simulink model "control_core"  (R2022b)
settings: Solver=FixedStepAuto  StartTime=0.0  StopTime=60  FixedStep=.01  RelTol=1e-3
undefined symbols (not defined in the file): CdProp, Ct, Earth, g, Ixx, Iyy, Izz, larm, mass, WGS84
libraries: slpidlib x6, sharedtransform x4, simulink x2, aerolibutil x2, aerolibtransform2 x1, shared6dof x1, aerolibfltsims x1, vrlib x1
(part 1 of 2)
settings Model: Creator=aaron  LastModifiedBy=aaron
settings DebuggingCC: ModelReferenceExtraNoncontSigs=none

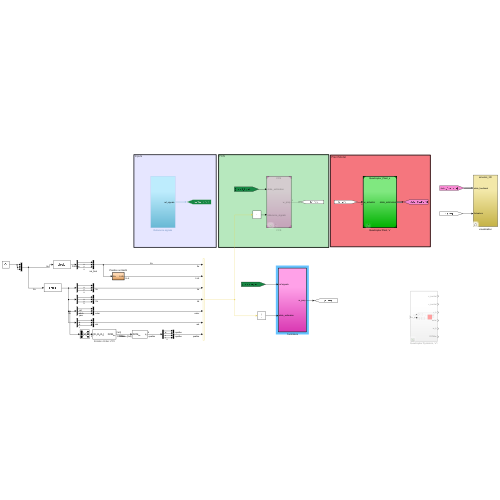
[thumbnail: Simulink's stored preview of the top-level diagram]
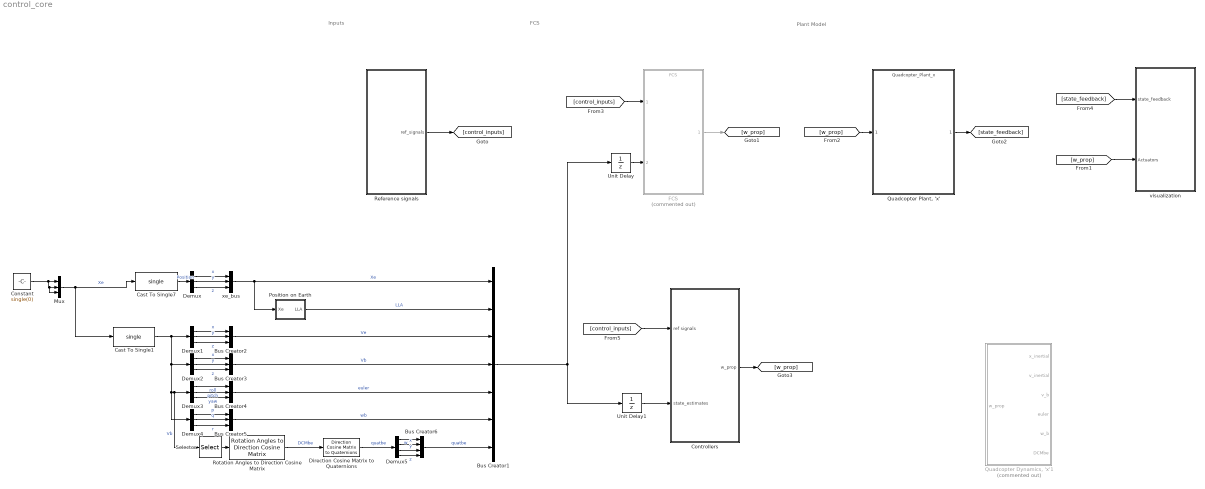
== system control_core ==
  note: Plant Model
  note: Inputs
  note: FCS
  Bus Creator1 : BusCreator  Inputs=7  OutDataTypeStr=Bus: state_estimates
  Bus Creator2 : BusCreator  Inputs=3  OutDataTypeStr=Bus: Velocity
  Bus Creator3 : BusCreator  Inputs=3  OutDataTypeStr=Bus: Velocity
  Bus Creator4 : BusCreator  Inputs=3  OutDataTypeStr=Bus: euler
  Bus Creator5 : BusCreator  Inputs=3  OutDataTypeStr=Bus: body_rates
  Bus Creator6 : BusCreator  Inputs=4  OutDataTypeStr=Bus: quat
  Cast To Single1 : DataTypeConversion  OutDataTypeStr=single  SaturateOnIntegerOverflow=off  RndMeth=Floor
  Cast To Single7 : DataTypeConversion  OutDataTypeStr=single  SaturateOnIntegerOverflow=off  RndMeth=Floor
  Constant : Constant  Value=single(0)  OutDataTypeStr=single
  Controllers : Subsystem  TreatAsAtomicUnit=on
  Demux{,1..4} (5 alike) : Demux  Outputs=3
  Demux5 : Demux
  Direction Cosine Matrix to Quaternions : sharedtransform/Direction Cosine Matrix  to Quaternions  aMode=0  action=None  tolerance=eps(2)
      settings: LibrarySourceBlock=|
      | aerolibtransform2/Direction Cosine Matrix
      | to Quaternions
  FCS : ModelReference  Commented=on  ModelNameDialog=FCS  SimulationMode=Normal  ModelReferenceVersion=1.59
  Mux : Mux  Inputs=3
  Position on Earth : Subsystem  Priority=1  TreatAsAtomicUnit=on
  "Quadcopter Dynamics, 'x'1" : Subsystem  Commented=on
  "Quadcopter Plant, 'x'" : ModelReference  ModelNameDialog=Quadcopter_Plant_x  SimulationMode=Normal  ModelReferenceVersion=1.62
  Reference signals : Subsystem
  Rotation Angles to Direction Cosine Matrix : sharedtransform/Rotation Angles to Direction Cosine Matrix  rotationOrder=ZYX  aMode=aMode
  Selector : Selector  InputPortWidth=3  IndexOptions=Index vector (dialog)  Indices=[3 2 1]  OutputSizes=1
  Unit Delay : UnitDelay  SampleTime=-1  HasFrameUpgradeWarning=on
  Unit Delay1 : UnitDelay  SampleTime=-1  HasFrameUpgradeWarning=on
  visualization : Subsystem  Variant=on  VariantControl=Choice
  xe_bus : BusCreator  Inputs=3  OutDataTypeStr=Bus: Position
  wires:
  FCS/1 -> [w_prop]
  Bus Creator1/1 -> Unit Delay/1, Unit Delay1/1
  Unit Delay/1 -> FCS/2
  [w_prop] -> visualization/2(Actuators)
  [w_prop] -> "Quadcopter Plant, 'x'"/1
  Reference signals/1(ref_signals) -> [control_inputs]
  [control_inputs] -> FCS/1
  "Quadcopter Plant, 'x'"/1 -> [state_feedback]
  [state_feedback] -> visualization/1(state_feedback)
  Demux4/2 -> Bus Creator5/2  "q"
  Demux5/4 -> Bus Creator6/4  "z"
  Demux/2 -> xe_bus/2  "y"
  Demux/3 -> xe_bus/3  "z"
  xe_bus/1 -> Bus Creator1/1, Position on Earth/1(Xe)  "Xe"
  Bus Creator4/1 -> Bus Creator1/5  "euler"
  Direction Cosine Matrix to Quaternions/1 -> Demux5/1  "quatbe"
  Demux/1 -> xe_bus/1  "x"
  Demux1/3 -> Bus Creator2/3  "z"
  Demux1/2 -> Bus Creator2/2  "y"
  Demux1/1 -> Bus Creator2/1  "x"
  Demux3/1 -> Bus Creator4/1  "roll"
  Demux3/2 -> Bus Creator4/2  "pitch"
  Demux3/3 -> Bus Creator4/3  "yaw"
  Bus Creator2/1 -> Bus Creator1/3  "Ve"
  Demux2/2 -> Bus Creator3/2  "y"
  Demux2/1 -> Bus Creator3/1  "x"
  Mux/1 -> Cast To Single1/1, Cast To Single7/1  "Xe"
  Demux4/1 -> Bus Creator5/1  "p"
  Bus Creator5/1 -> Bus Creator1/6  "wb"
  Bus Creator6/1 -> Bus Creator1/7  "quatbe"
  Demux2/3 -> Bus Creator3/3  "z"
  Demux5/3 -> Bus Creator6/3  "y"
  Bus Creator3/1 -> Bus Creator1/4  "Vb"
  Demux4/3 -> Bus Creator5/3  "r"
  Rotation Angles to Direction Cosine Matrix/1 -> Direction Cosine Matrix to Quaternions/1  "DCMbe"
  Selector/1 -> Rotation Angles to Direction Cosine Matrix/1
  Position on Earth/1(LLA) -> Bus Creator1/2  "LLA"
  Demux5/1 -> Bus Creator6/1  "w"
  Demux5/2 -> Bus Creator6/2  "x"
  Constant/1 -> Mux/3, Mux/2, Mux/1
  Cast To Single7/1 -> Demux/1  "Position"
  Cast To Single1/1 -> Demux4/1, Selector/1, Demux3/1, Demux2/1, Demux1/1  "Vb"
  [control_inputs] -> Controllers/1(ref signals)
  Unit Delay1/1 -> Controllers/2(state_estimates)
  Controllers/1(w_prop) -> [w_prop]

== system control_core/Controllers ==
  ref signals : Inport  OutDataTypeStr=Bus: reference_signals  LockScale=on
  state_estimates : Inport  Port=2  OutDataTypeStr=Bus: state_estimates  LockScale=on
  Flight Controller : Subsystem
  Motor Mixing : Subsystem
  w_prop : Outport
  wires:
  state_estimates/1 -> Flight Controller/2(state_estimates)
  Flight Controller/1(Force command) -> Motor Mixing/1(Force)
  Motor Mixing/1(motor_rpm) -> w_prop/1  "w_prop"
  Flight Controller/2(Torque command) -> Motor Mixing/2(Torque)
  ref signals/1 -> Flight Controller/1(ref signals)

== system control_core/Position on Earth ==
  Xe : Inport  OutDataTypeStr=Bus: Position  Unit=m
  Bus Creator : BusCreator  Inputs=3  OutDataTypeStr=Bus: LLA
  Bus Selector : BusSelector  OutputSignals=x,y,z  OutputAsBus=on
  Bus to Vector : BusToVector
  Cast To Single : DataTypeConversion  OutDataTypeStr=single  SaturateOnIntegerOverflow=off  RndMeth=Floor
  Cast To Single1 : DataTypeConversion  OutDataTypeStr=single  SaturateOnIntegerOverflow=off  RndMeth=Floor
  Demux : Demux  Outputs=2
  Flat Earth to LLA : aerolibtransform2/Flat Earth to LLA  units=Metric (MKS)  ptype=Earth (WGS84)  F=1/298.257223563  R=6378137  refPosPort=off  LL0=[-122.389977, 37.615223]  psi=0
  href : Constant  Value=-4
  LLA : Outport  OutDataTypeStr=Bus: LLA  VectorParamsAs1DForOutWhenUnconnected=off
  wires:
  Bus Creator/1 -> LLA/1
  href/1 -> Flat Earth to LLA/2
  Demux/2 -> Bus Creator/2  "long"
  Flat Earth to LLA/1 -> Cast To Single/1
  Demux/1 -> Bus Creator/1  "lat"
  Flat Earth to LLA/2 -> Cast To Single1/1  "altitude"
  Xe/1 -> Bus Selector/1
  Bus Selector/1 -> Bus to Vector/1
  Bus to Vector/1 -> Flat Earth to LLA/1
  Cast To Single/1 -> Demux/1
  Cast To Single1/1 -> Bus Creator/3  "altitude"

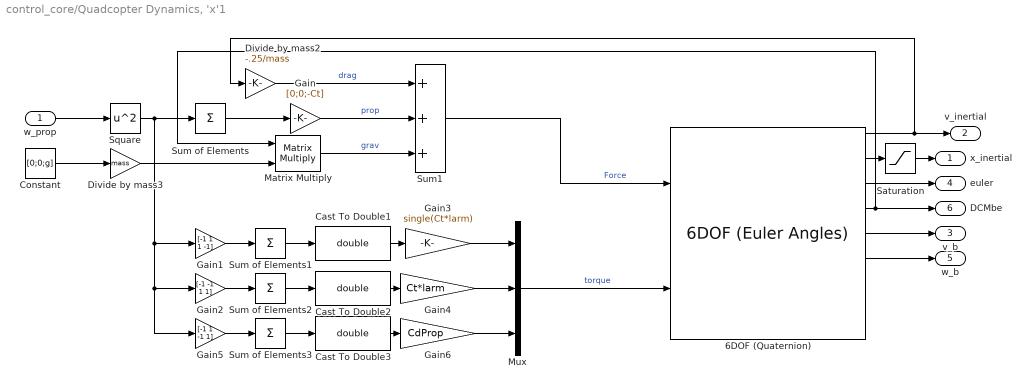
== system control_core/Quadcopter Dynamics, 'x'1 ==
  w_prop : Inport
  6DOF (Quaternion) : shared6dof/6DOF (Euler Angles)  units=Metric (MKS)  mtype=Fixed  rep=Euler Angles  xme_0=[0,0,0]  Vm_0=[0,0,0]  eul_0=[0,0,0]  pm_0=[0,0,0]  mass_0=mass  mass_e=0.5  mass_f=2.0  inertia=diag([Ixx Iyy Izz])  inertia_e=eye(3)  inertia_f=2*eye(3)  k_quat=Vehicle.SixDOF.quatGain  vre_flag=on  abi_flag=on  aMode=aMode  xme_statename=''  Vm_statename=''  eul_statename=''  quat_statename=''  pm_statename=''  mass_statename=''
  Cast To Double1 : DataTypeConversion  OutDataTypeStr=double  SaturateOnIntegerOverflow=off  RndMeth=Floor
  Cast To Double2 : DataTypeConversion  OutDataTypeStr=double  SaturateOnIntegerOverflow=off  RndMeth=Floor
  Cast To Double3 : DataTypeConversion  OutDataTypeStr=double  SaturateOnIntegerOverflow=off  RndMeth=Floor
  Constant : Constant  Value=[0;0;g]
  Divide by mass2 : Gain  Gain=-.25/mass
  Divide by mass3 : Gain  Gain=mass
  Gain : Gain  Gain=[0;0;-Ct]
  Gain1 : Gain  Gain=[-1 1 1 -1]
  Gain2 : Gain  Gain=[-1 -1 1 1]
  Gain3 : Gain  Gain=single(Ct*larm)
  Gain4 : Gain  Gain=Ct*larm
  Gain5 : Gain  Gain=[-1 1 -1 1]
  Gain6 : Gain  Gain=CdProp
  Matrix Multiply : Product  Multiplication=Matrix(*)
  Mux : Mux  Inputs=3
  Saturation : Saturate  UpperLimit=[inf inf 0]  LowerLimit=-inf
  Square : Math  Operator=square
  Sum of Elements{,1..3} (4 alike) : Sum  Inputs=+
  Sum1 : Sum  Inputs=+++
  x_inertial : Outport
  v_inertial : Outport  Port=2
  v_b : Outport  Port=3
  euler : Outport  Port=4
  w_b : Outport  Port=5
  DCMbe : Outport  Port=6
  wires:
  Sum1/1 -> 6DOF (Quaternion)/1  "Force"
  Constant/1 -> Divide by mass3/1
  6DOF (Quaternion)/1 -> v_inertial/1, Divide by mass2/1
  Divide by mass2/1 -> Sum1/1  "drag"
  w_prop/1 -> Square/1
  Square/1 -> Gain5/1, Gain2/1, Gain1/1, Sum of Elements/1
  Sum of Elements/1 -> Gain/1
  Gain/1 -> Sum1/2  "prop"
  Gain1/1 -> Sum of Elements1/1
  Gain2/1 -> Sum of Elements2/1
  Gain5/1 -> Sum of Elements3/1
  Gain3/1 -> Mux/1
  Gain4/1 -> Mux/2
  Gain6/1 -> Mux/3
  Mux/1 -> 6DOF (Quaternion)/2  "torque"
  6DOF (Quaternion)/5 -> v_b/1
  6DOF (Quaternion)/2 -> Saturation/1
  6DOF (Quaternion)/6 -> w_b/1
  6DOF (Quaternion)/3 -> euler/1
  6DOF (Quaternion)/4 -> Matrix Multiply/1, DCMbe/1
  Cast To Double1/1 -> Gain3/1
  Sum of Elements1/1 -> Cast To Double1/1
  Cast To Double2/1 -> Gain4/1
  Sum of Elements2/1 -> Cast To Double2/1
  Sum of Elements3/1 -> Cast To Double3/1
  Cast To Double3/1 -> Gain6/1
  Saturation/1 -> x_inertial/1
  Divide by mass3/1 -> Matrix Multiply/2
  Matrix Multiply/1 -> Sum1/3  "grav"

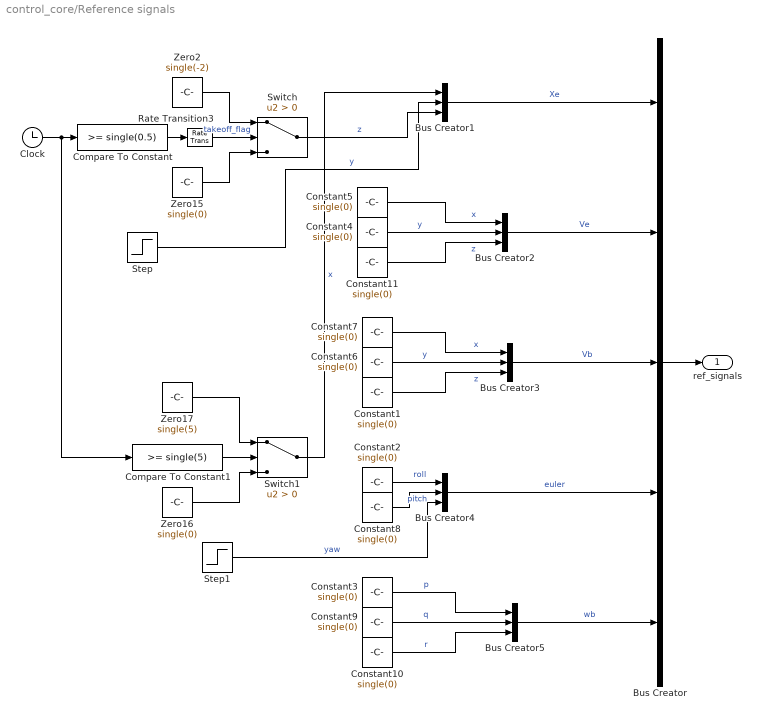
== system control_core/Reference signals ==
  Bus Creator : BusCreator  Inputs=5  OutDataTypeStr=Bus: reference_signals
      settings: InheritFromInputs=off
  Bus Creator1 : BusCreator  Inputs=3  OutDataTypeStr=Bus: Position
  Bus Creator2 : BusCreator  Inputs=3  OutDataTypeStr=Bus: Velocity
  Bus Creator3 : BusCreator  Inputs=3  OutDataTypeStr=Bus: Velocity
  Bus Creator4 : BusCreator  Inputs=3  OutDataTypeStr=Bus: euler
  Bus Creator5 : BusCreator  Inputs=3  OutDataTypeStr=Bus: body_rates
  Clock : Clock
  Compare To Constant : simulink/Logic and Bit Operations/Compare To Constant  relop=>=  const=single(0.5)  OutDataTypeStr=boolean
  Compare To Constant1 : simulink/Logic and Bit Operations/Compare To Constant  relop=>=  const=single(5)  OutDataTypeStr=boolean
  Constant{1..11} (11 alike) : Constant  Value=single(0)  OutDataTypeStr=single
  Rate Transition3 : RateTransition  OutPortSampleTime=.01
  Step : Step  Time=10  After=single(5)  OutDataTypeStr=single  SampleTime=0
  Step1 : Step  Time=10  After=single(pi/2)  OutDataTypeStr=single  SampleTime=0
  Switch : Switch  Criteria=u2 > Threshold  SaturateOnIntegerOverflow=off  InputSameDT=off
  Switch1 : Switch  Criteria=u2 > Threshold  SaturateOnIntegerOverflow=off  InputSameDT=off
  Zero15 : Constant  Value=single(0)  OutDataTypeStr=single
  Zero16 : Constant  Value=single(0)  OutDataTypeStr=single
  Zero17 : Constant  Value=single(5)  OutDataTypeStr=single
  Zero2 : Constant  Value=single(-2)  OutDataTypeStr=single
  ref_signals : Outport  OutDataTypeStr=Bus: reference_signals  SampleTime=.01  LockScale=on
  wires:
  Bus Creator4/1 -> Bus Creator/4  "euler"
  Bus Creator1/1 -> Bus Creator/1  "Xe"
  Bus Creator2/1 -> Bus Creator/2  "Ve"
  Bus Creator/1 -> ref_signals/1
  Zero15/1 -> Switch/3
  Zero2/1 -> Switch/1
  Clock/1 -> Compare To Constant1/1, Compare To Constant/1
  Compare To Constant/1 -> Rate Transition3/1
  Rate Transition3/1 -> Switch/2  "takeoff_flag"
  Compare To Constant1/1 -> Switch1/2
  Zero16/1 -> Switch1/3
  Zero17/1 -> Switch1/1
  Switch/1 -> Bus Creator1/3  "z"
  Step/1 -> Bus Creator1/2  "y"
  Step1/1 -> Bus Creator4/3  "yaw"
  Switch1/1 -> Bus Creator1/1  "x"
  Constant2/1 -> Bus Creator4/1  "roll"
  Constant5/1 -> Bus Creator2/1  "x"
  Constant4/1 -> Bus Creator2/2  "y"
  Constant11/1 -> Bus Creator2/3  "z"
  Constant7/1 -> Bus Creator3/1  "x"
  Bus Creator3/1 -> Bus Creator/3  "Vb"
  Constant6/1 -> Bus Creator3/2  "y"
  Constant1/1 -> Bus Creator3/3  "z"
  Constant8/1 -> Bus Creator4/2  "pitch"
  Constant9/1 -> Bus Creator5/2  "q"
  Constant10/1 -> Bus Creator5/3  "r"
  Bus Creator5/1 -> Bus Creator/5  "wb"
  Constant3/1 -> Bus Creator5/1  "p"

== system control_core/visualization ==
  state_feedback : Inport  OutDataTypeStr=Bus: state_estimates
  Actuators : Inport  Port=2
  flight_gear : Subsystem  VariantControl=sim_3D == 0
  simulink_3D : Subsystem  VariantControl=sim_3D == 1

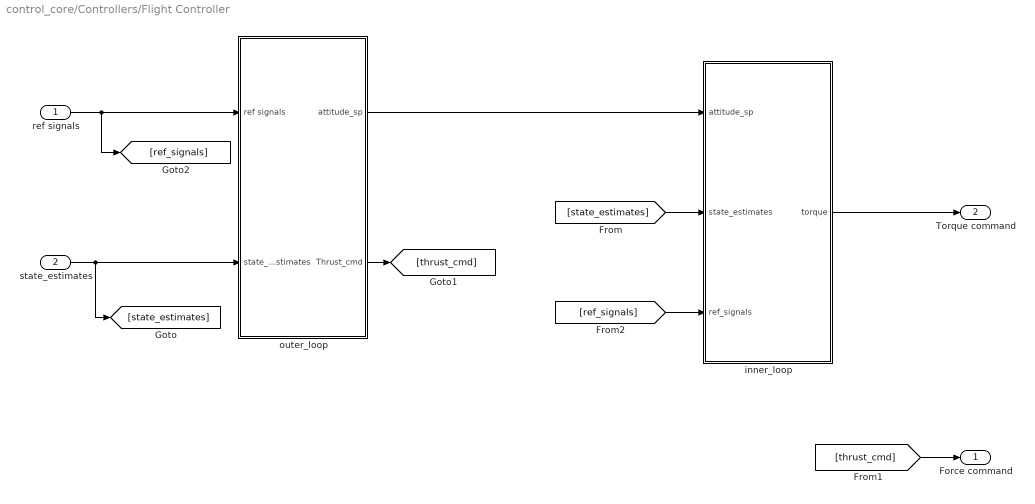
== system control_core/Controllers/Flight Controller ==
  ref signals : Inport  OutDataTypeStr=Bus: reference_signals  LockScale=on
  state_estimates : Inport  Port=2  OutDataTypeStr=Bus: state_estimates  LockScale=on
  inner_loop : Subsystem
  outer_loop : Subsystem
  Force command : Outport
  Torque command : Outport  Port=2
  wires:
  [ref_signals] -> inner_loop/3(ref_signals)
  [thrust_cmd] -> Force command/1
  outer_loop/2(Thrust_cmd) -> [thrust_cmd]
  inner_loop/1(torque) -> Torque command/1
  [state_estimates] -> inner_loop/2(state_estimates)
  outer_loop/1(attitude_sp) -> inner_loop/1(attitude_sp)
  ref signals/1 -> outer_loop/1(ref signals), [ref_signals]
  state_estimates/1 -> [state_estimates], outer_loop/2(state_estimates)

== system control_core/Controllers/Motor Mixing ==
  Force : Inport
  Torque : Inport  Port=2
  Cast To Single : DataTypeConversion  OutDataTypeStr=single  SaturateOnIntegerOverflow=off  RndMeth=Floor
  MATLAB Function : MATLAB Function  TreatAsAtomicUnit=on
  Matrix Multiply : Product  Multiplication=Matrix(*)
  Mux : Mux  Inputs=2
  Saturation : Saturate  UpperLimit=2000  LowerLimit=0
  SignedSqrt1 : Sqrt  Operator=signedSqrt  IntermediateResultsDataTypeStr=single
  motor_rpm : Outport
  wires:
  Mux/1 -> Cast To Single/1
  Cast To Single/1 -> Matrix Multiply/2
  MATLAB Function/1(controlMatInv) -> Matrix Multiply/1  "invcontrolMat"
  Matrix Multiply/1 -> SignedSqrt1/1
  SignedSqrt1/1 -> Saturation/1
  Saturation/1 -> motor_rpm/1
  Force/1 -> Mux/1
  Torque/1 -> Mux/2  "torque"

== system control_core/visualization/flight_gear ==
  state_feedback : Inport  OutDataTypeStr=Bus: state_estimates
  Actuators : Inport  Port=2
  Flight_gear : Subsystem
  wires:
  state_feedback/1 -> [state_feedback]
  [state_feedback] -> Flight_gear/1(state_feedback)
  Actuators/1 -> [actuators]

== system control_core/visualization/simulink_3D ==
  state_feedback : Inport  OutDataTypeStr=Bus: state_estimates
  Actuators : Inport  Port=2
  Simulink 3D : Subsystem  VariantControl=VSS_VISUALIZATION==VisualizationMode.Simulink_3D
  wires:
  state_feedback/1 -> [state_feedback]
  [state_feedback] -> Simulink 3D/1(state_feedback)
  Actuators/1 -> [actuators]
  [actuators] -> Simulink 3D/2(Actuators)

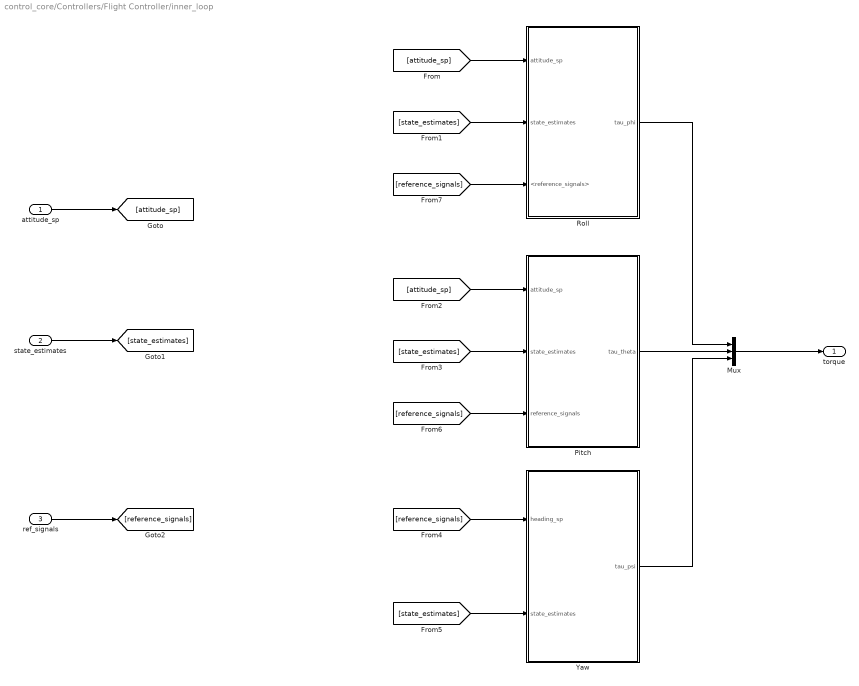
== system control_core/Controllers/Flight Controller/inner_loop ==
  attitude_sp : Inport
  state_estimates : Inport  Port=2  OutDataTypeStr=Bus: state_estimates
  ref_signals : Inport  Port=3  OutDataTypeStr=Bus: reference_signals
  Mux : Mux  Inputs=3
  Pitch : Subsystem
  Roll : Subsystem
  Yaw : Subsystem
  torque : Outport
  wires:
  Yaw/1(tau_psi) -> Mux/3
  Pitch/1(tau_theta) -> Mux/2
  Mux/1 -> torque/1
  Roll/1(tau_phi) -> Mux/1
  [state_estimates] -> Yaw/2(state_estimates)
  [state_estimates] -> Pitch/2(state_estimates)
  [attitude_sp] -> Pitch/1(attitude_sp)
  [state_estimates] -> Roll/2(state_estimates)
  [attitude_sp] -> Roll/1(attitude_sp)
  state_estimates/1 -> [state_estimates]
  attitude_sp/1 -> [attitude_sp]
  ref_signals/1 -> [reference_signals]
  [reference_signals] -> Yaw/1(heading_sp)
  [reference_signals] -> Pitch/3(reference_signals)
  [reference_signals] -> Roll/3(<reference_signals>)

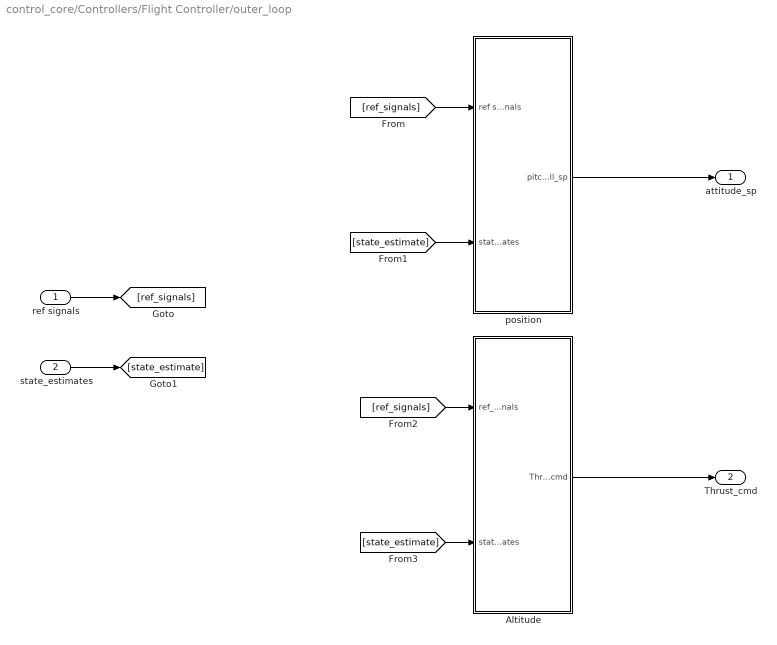
== system control_core/Controllers/Flight Controller/outer_loop ==
  ref signals : Inport  OutDataTypeStr=Bus: reference_signals  LockScale=on
  state_estimates : Inport  Port=2  OutDataTypeStr=Bus: state_estimates  LockScale=on
  Altitude : Subsystem
  position : Subsystem
  attitude_sp : Outport
  Thrust_cmd : Outport  Port=2
  wires:
  [state_estimate] -> Altitude/2(state_estimates)
  [ref_signals] -> Altitude/1(ref_signals)
  [state_estimate] -> position/2(state_estimates)
  [ref_signals] -> position/1(ref signals)
  state_estimates/1 -> [state_estimate]
  ref signals/1 -> [ref_signals]
  Altitude/1(Thrust_cmd) -> Thrust_cmd/1
  position/1(pitch_roll_sp) -> attitude_sp/1

== system control_core/visualization/flight_gear/Flight_gear ==
  state_feedback : Inport  OutDataTypeStr=Bus: state_estimates
  Bus Selector : BusSelector  OutputSignals=LLA,euler
  Demux5 : Demux  Outputs=3
  FlightGear Preconfigured 6DoF Animation : aerolibfltsims/FlightGear Preconfigured 6DoF Animation  Commented=on  xFlightGearVersion=v2019.1  DestinationIpAddress=127.0.0.1  DestinationPort=5502  SampleTime=.0001  packetVersion=24
  Mux1 : Mux  Inputs=2
  Mux2 : Mux  Inputs=3
  Transpose : Math  Operator=transpose
  wires:
  Demux5/3 -> Mux2/3
  Mux2/1 -> Transpose/1
  Demux5/2 -> Mux2/1
  Mux1/1 -> FlightGear Preconfigured 6DoF Animation/1
  Bus Selector/2 -> Mux1/2  "<euler>"
  Demux5/1 -> Mux2/2
  Transpose/1 -> Mux1/1
  Bus Selector/1 -> Demux5/1  "<LLA>"
  state_feedback/1 -> Bus Selector/1

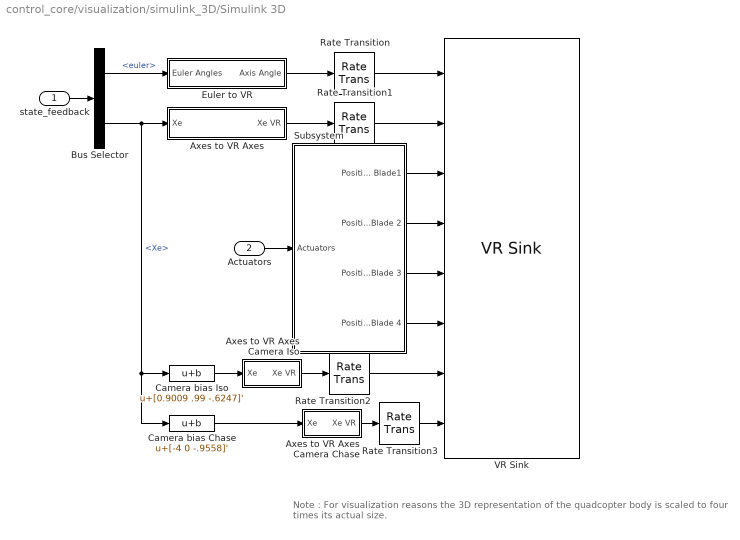
== system control_core/visualization/simulink_3D/Simulink 3D ==
  note: Note : For visualization reasons the 3D representation of the quadcopter body is scaled to four times its actual size.
  state_feedback : Inport  OutDataTypeStr=Bus: state_estimates
  Actuators : Inport  Port=2
  Axes to VR Axes : Subsystem
  Axes to VR Axes Camera Chase : Subsystem
  Axes to VR Axes Camera Iso : Subsystem
  Bus Selector : BusSelector  OutputSignals=euler,Xe
  Camera bias Chase : Bias  Bias=[-4 0 -.9558]'  SaturateOnIntegerOverflow=off
  Camera bias Iso : Bias  Bias=[0.9009 .99 -.6247]'  SaturateOnIntegerOverflow=off
  Euler to VR : Subsystem
  Rate Transition{,1..3} (4 alike) : RateTransition
  Subsystem : Subsystem
  VR Sink : vrlib/VR Sink  InstantiateOnLoad=on  SampleTime=10*.01  ViewEnable=on  RemoteChange=off  RemoteView=off  FieldsWritten=QuadBody.rotation.4.1.1.double#QuadBody.translation.3.1.1.double#Blade1.rotation.4.1.1.double#Blade2.rotation.4.1.1.double#Blade3.rotation.4.1.1.double#Blade4.rotation.4.1.1.double#IsoNoRotation.position.3.1.1.double#OnQuadNoRotation.position.3.1.1.double  WorldFileName=asbQuadcopterWorld.wrl  AutoView=on  VideoDimensions=[]  AllowVariableSize=off  FigureProperties="{'Position', 'Name', 'Viewpoint', 'CameraBound', 'CameraDirection', 'CameraPosition', 'CameraUpVector', 'ZoomFactor', 'Antialiasing', 'Headlight', 'Lighting', 'NavPanel', 'Sound', 'StatusBar', 'Stereo3D', 'Stereo3DCameraOffset', 'Stereo3DHIT', 'ToolBar', 'Textures', 'Transparency', 'Triad', 'Wireframe', 'NavZones', 'NavMode', 'NavSpeed', 'CaptureFileFormat', 'CaptureFileName', 'Record2DCompressMethod', 'Record2DCompressQuality', 'Record2D', 'Record2DFileName', 'Record2DFPS'; [5.0000000000000000e+00   9.2000000000000000e+01   5.7600000000000000e+02   3.5000000000000000e+02], '', 'Isometric', 'on', [0.0000000000000000e+00   0.0000000000000000e+00  -1.0000000000000000e+00], [0.0000000000000000e+00   0.0000000000000000e+00   0.0000000000000000e+00], [0.0000000000000000e+00   1.0000000000000000e+00   0.0000000000000000e+00], [1.0000000000000000e+00], 'off', 'on', 'on', 'halfbar', 'on', 'on', 'off', [1.0000000149011612e-01], [0.0000000000000000e+00], 'on', 'on', 'on', 'none', 'off', 'off', 'fly', 'normal', 'tif', '%f_anim_%n.tif', 'auto', [7.5000000000000000e+01], 'off', '%f_anim_%n.avi', 'auto'}"
  wires:
  Euler to VR/1(Axis Angle) -> Rate Transition/1
  Axes to VR Axes/1(Xe VR) -> Rate Transition1/1
  Bus Selector/1 -> Euler to VR/1(Euler Angles)  "<euler>"
  Bus Selector/2 -> Axes to VR Axes/1(Xe), Camera bias Chase/1, Camera bias Iso/1  "<Xe>"
  state_feedback/1 -> Bus Selector/1
  Actuators/1 -> Subsystem/1(Actuators)
  Axes to VR Axes Camera Iso/1(Xe VR) -> Rate Transition2/1
  Camera bias Iso/1 -> Axes to VR Axes Camera Iso/1(Xe)
  Rate Transition/1 -> VR Sink/1
  Rate Transition1/1 -> VR Sink/2
  Subsystem/1(Position Blade1) -> VR Sink/3
  Subsystem/2(Position Blade 2) -> VR Sink/4
  Subsystem/3(Position Blade 3) -> VR Sink/5
  Subsystem/4(Position Blade 4) -> VR Sink/6
  Rate Transition2/1 -> VR Sink/7
  Axes to VR Axes Camera Chase/1(Xe VR) -> Rate Transition3/1
  Rate Transition3/1 -> VR Sink/8
  Camera bias Chase/1 -> Axes to VR Axes Camera Chase/1(Xe)

== system control_core/Controllers/Flight Controller/inner_loop/Pitch ==
  attitude_sp : Inport
  state_estimates : Inport  Port=2  OutDataTypeStr=Bus: state_estimates
  reference_signals : Inport  Port=3  OutDataTypeStr=Bus: reference_signals
  Bus Selector : BusSelector  OutputSignals=euler.pitch
  PID Controller : slpidlib/PID Controller  Controller=PID  Form=Parallel  TimeDomain=Discrete-time  UseExternalTs=off  SampleTime=-1  IntegratorMethod=Forward Euler  FilterMethod=Forward Euler  ControllerParametersSource=internal  P=0.000755  I=1.95e-05  UseKiTs=off  D=0.00509  N=1.0382  UseFilter=on  TunerSelectOption=Transfer Function Based (PID Tuner App)  InitialConditionSource=internal  InitialConditionForIntegrator=0  InitialConditionForFilter=0  DifferentiatorICPrevScaledInput=0  ExternalReset=none  TrackingMode=off  Kt=1  LimitOutput=off  SatLimitsSource=internal  UpperSaturationLimit=inf  LowerSaturationLimit=-inf  LinearizeAsGain=on  AntiWindupMode=clamping  Kb=1  LimitIntegrator=off  UpperIntegratorSaturationLimit=inf  LowerIntegratorSaturationLimit=-inf  POutMin=[]  POutMax=[]  IOutMin=[]  IOutMax=[]  DOutMin=[]  DOutMax=[]  NOutMin=[]  NOutMax=[]  SumOutMin=[]  SumOutMax=[]  SaturationOutMin=[]  SaturationOutMax=[]  PParamMin=[]  PParamMax=[]  IParamMin=[]  IParamMax=[]  DParamMin=[]  DParamMax=[]  NParamMin=[]  NParamMax=[]  KbParamMin=[]  KbParamMax=[]  KtParamMin=[]  KtParamMax=[]  KbOutMin=[]  KbOutMax=[]  KtOutMin=[]  KtOutMax=[]  IntegratorOutMin=[]  IntegratorOutMax=[]  FilterOutMin=[]  FilterOutMax=[]  SumI1OutMin=[]  SumI1OutMax=[]  SumI2OutMin=[]  SumI2OutMax=[]  SumI3OutMin=[]  SumI3OutMax=[]  SumI4OutMin=[]  SumI4OutMax=[]  SumDOutMin=[]  SumDOutMax=[]  DifferentiatorOutMin=[]  DifferentiatorOutMax=[]  FilterDiffOutCoefMin=[]  FilterDiffOutCoefMax=[]  ReciprocalOutMin=[]  ReciprocalOutMax=[]  SumDenOutMin=[]  SumDenOutMax=[]  SumNumOutMin=[]  SumNumOutMax=[]  DivideOutMin=[]  DivideOutMax=[]  UdiffTsProdOutMin=[]  UdiffTsProdOutMax=[]  NTsProdOutMin=[]  NTsProdOutMax=[]  UintegralTsProdOutMin=[]  UintegralTsProdOutMax=[]  UngainTsProdOutMin=[]  UngainTsProdOutMax=[]  ClampingZeroOutDataTypeStr=Inherit: Inherit via back propagation  ClampingZeroOutMin=[]  ClampingZeroOutMax=[]  FilterDenConstantOutDataTypeStr=Inherit: Inherit via back propagation  FilterDenConstantOutMin=[]  FilterDenConstantOutMax=[]  PCopyOutDataTypeStr=Inherit: Inherit via back propagation  PCopyOutMin=[]  PCopyOutMax=[]  NCopyOutDataTypeStr=Inherit: Inherit via back propagation  NCopyOutMin=[]  NCopyOutMax=[]  IntegratorContinuousStateAttributes=''  IntegratorStateMustResolveToSignalObject=off  IntegratorRTWStateStorageClass=Auto  FilterContinuousStateAttributes=''  FilterStateMustResolveToSignalObject=off  FilterRTWStateStorageClass=Auto  ParallelPVariant=InternalParameters  IdealPVariant=Disabled  IVariant=InternalParameters  DVariant=InternalParameters  IntegratorVariant=Discrete  SatVariant=Disabled  AWVariant=Passthrough  PCopyVariant=Disabled  TRVariant=Disabled  FdbkBlocksVariant=Forward  IdealPFdbkVariant=Disabled  SatFdbkVariant=Disabled  DerivativeFilterVariant=ForwardEulerFilter  NVariant=InternalParameters  NCopyVariant=Disabled  FilterICVariant=InternalICsFilter  IntegratorICVariant=InternalICs  ExternalResetVariant=Disabled  TRSumVariant=Passthrough  SumFdbkVariant=Disabled  SumVariant=Sum_PID  TsampFilterVariant=InternalTs  TsampNgainVariant=Passthrough  TsampIntegralVariant=Passthrough  ExternalSaturationOutDataTypeStr=Inherit: Same as second input
  Selector : Selector  InputPortWidth=2  IndexOptions=Index vector (dialog)  Indices=[2]  OutputSizes=1
  Sum : Sum  Inputs=|+-
  Terminator : Terminator
  tau_theta : Outport
  wires:
  Selector/1 -> Sum/1
  reference_signals/1 -> Terminator/1
  state_estimates/1 -> Bus Selector/1
  Bus Selector/1 -> Sum/2  "<pitch>"
  PID Controller/1 -> tau_theta/1
  Sum/1 -> PID Controller/1
  attitude_sp/1 -> Selector/1

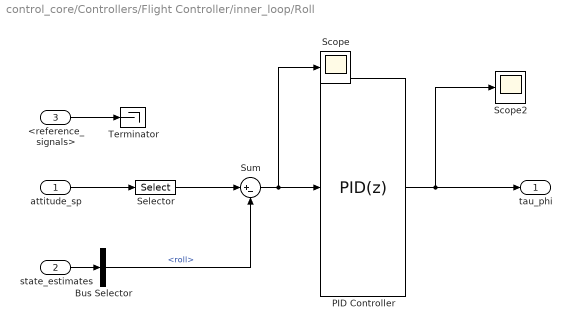
== system control_core/Controllers/Flight Controller/inner_loop/Roll ==
  attitude_sp : Inport
  state_estimates : Inport  Port=2  OutDataTypeStr=Bus: state_estimates
  <reference_signals> : Inport  Port=3  OutDataTypeStr=Bus: reference_signals
  Bus Selector : BusSelector  OutputSignals=euler.roll
  PID Controller : slpidlib/PID Controller  Controller=PID  Form=Parallel  TimeDomain=Discrete-time  UseExternalTs=off  SampleTime=-1  IntegratorMethod=Forward Euler  FilterMethod=Forward Euler  ControllerParametersSource=internal  P=0.00222776202264695  I=2.18485015437245e-05  UseKiTs=off  D=0.0134340999324703  N=1.24748629813611  UseFilter=on  TunerSelectOption=Transfer Function Based (PID Tuner App)  InitialConditionSource=internal  InitialConditionForIntegrator=0  InitialConditionForFilter=0  DifferentiatorICPrevScaledInput=0  ExternalReset=none  TrackingMode=off  Kt=1  LimitOutput=off  SatLimitsSource=internal  UpperSaturationLimit=inf  LowerSaturationLimit=-inf  LinearizeAsGain=on  AntiWindupMode=clamping  Kb=1  LimitIntegrator=off  UpperIntegratorSaturationLimit=inf  LowerIntegratorSaturationLimit=-inf  POutMin=[]  POutMax=[]  IOutMin=[]  IOutMax=[]  DOutMin=[]  DOutMax=[]  NOutMin=[]  NOutMax=[]  SumOutMin=[]  SumOutMax=[]  SaturationOutMin=[]  SaturationOutMax=[]  PParamMin=[]  PParamMax=[]  IParamMin=[]  IParamMax=[]  DParamMin=[]  DParamMax=[]  NParamMin=[]  NParamMax=[]  KbParamMin=[]  KbParamMax=[]  KtParamMin=[]  KtParamMax=[]  KbOutMin=[]  KbOutMax=[]  KtOutMin=[]  KtOutMax=[]  IntegratorOutMin=[]  IntegratorOutMax=[]  FilterOutMin=[]  FilterOutMax=[]  SumI1OutMin=[]  SumI1OutMax=[]  SumI2OutMin=[]  SumI2OutMax=[]  SumI3OutMin=[]  SumI3OutMax=[]  SumI4OutMin=[]  SumI4OutMax=[]  SumDOutMin=[]  SumDOutMax=[]  DifferentiatorOutMin=[]  DifferentiatorOutMax=[]  FilterDiffOutCoefMin=[]  FilterDiffOutCoefMax=[]  ReciprocalOutMin=[]  ReciprocalOutMax=[]  SumDenOutMin=[]  SumDenOutMax=[]  SumNumOutMin=[]  SumNumOutMax=[]  DivideOutMin=[]  DivideOutMax=[]  UdiffTsProdOutMin=[]  UdiffTsProdOutMax=[]  NTsProdOutMin=[]  NTsProdOutMax=[]  UintegralTsProdOutMin=[]  UintegralTsProdOutMax=[]  UngainTsProdOutMin=[]  UngainTsProdOutMax=[]  ClampingZeroOutDataTypeStr=Inherit: Inherit via back propagation  ClampingZeroOutMin=[]  ClampingZeroOutMax=[]  FilterDenConstantOutDataTypeStr=Inherit: Inherit via back propagation  FilterDenConstantOutMin=[]  FilterDenConstantOutMax=[]  PCopyOutDataTypeStr=Inherit: Inherit via back propagation  PCopyOutMin=[]  PCopyOutMax=[]  NCopyOutDataTypeStr=Inherit: Inherit via back propagation  NCopyOutMin=[]  NCopyOutMax=[]  IntegratorContinuousStateAttributes=''  IntegratorStateMustResolveToSignalObject=off  IntegratorRTWStateStorageClass=Auto  FilterContinuousStateAttributes=''  FilterStateMustResolveToSignalObject=off  FilterRTWStateStorageClass=Auto  ParallelPVariant=InternalParameters  IdealPVariant=Disabled  IVariant=InternalParameters  DVariant=InternalParameters  IntegratorVariant=Discrete  SatVariant=Disabled  AWVariant=Passthrough  PCopyVariant=Disabled  TRVariant=Disabled  FdbkBlocksVariant=Forward  IdealPFdbkVariant=Disabled  SatFdbkVariant=Disabled  DerivativeFilterVariant=ForwardEulerFilter  NVariant=InternalParameters  NCopyVariant=Disabled  FilterICVariant=InternalICsFilter  IntegratorICVariant=InternalICs  ExternalResetVariant=Disabled  TRSumVariant=Passthrough  SumFdbkVariant=Disabled  SumVariant=Sum_PID  TsampFilterVariant=InternalTs  TsampNgainVariant=Passthrough  TsampIntegralVariant=Passthrough  ExternalSaturationOutDataTypeStr=Inherit: Same as second input
  Scope : Scope
  Scope2 : Scope
  Selector : Selector  InputPortWidth=2  IndexOptions=Index vector (dialog)  Indices=[1]  OutputSizes=1
  Sum : Sum  Inputs=|+-
  Terminator : Terminator
  tau_phi : Outport
  wires:
  Selector/1 -> Sum/1
  <reference_signals>/1 -> Terminator/1
  Bus Selector/1 -> Sum/2  "<roll>"
  state_estimates/1 -> Bus Selector/1
  PID Controller/1 -> tau_phi/1, Scope2/1
  Sum/1 -> Scope/1, PID Controller/1
  attitude_sp/1 -> Selector/1

== system control_core/Controllers/Flight Controller/inner_loop/Yaw ==
  heading_sp : Inport  OutDataTypeStr=Bus: reference_signals
  state_estimates : Inport  Port=2  OutDataTypeStr=Bus: state_estimates
  Bus Selector : BusSelector  OutputSignals=euler.yaw
  Bus Selector1 : BusSelector  OutputSignals=euler.yaw
  PID Controller : slpidlib/PID Controller  Controller=PD  Form=Parallel  TimeDomain=Discrete-time  UseExternalTs=off  SampleTime=-1  IntegratorMethod=Forward Euler  FilterMethod=Forward Euler  ControllerParametersSource=internal  P=0.00308709400862221  I=0  UseKiTs=off  D=0.020762699011989  N=9.31948574377754  UseFilter=on  TunerSelectOption=Transfer Function Based (PID Tuner App)  InitialConditionSource=internal  InitialConditionForIntegrator=0  InitialConditionForFilter=0  DifferentiatorICPrevScaledInput=0  ExternalReset=none  TrackingMode=off  Kt=1  LimitOutput=off  SatLimitsSource=internal  UpperSaturationLimit=inf  LowerSaturationLimit=-inf  LinearizeAsGain=on  AntiWindupMode=clamping  Kb=1  LimitIntegrator=off  UpperIntegratorSaturationLimit=inf  LowerIntegratorSaturationLimit=-inf  POutMin=[]  POutMax=[]  IOutMin=[]  IOutMax=[]  DOutMin=[]  DOutMax=[]  NOutMin=[]  NOutMax=[]  SumOutMin=[]  SumOutMax=[]  SaturationOutMin=[]  SaturationOutMax=[]  PParamMin=[]  PParamMax=[]  IParamMin=[]  IParamMax=[]  DParamMin=[]  DParamMax=[]  NParamMin=[]  NParamMax=[]  KbParamMin=[]  KbParamMax=[]  KtParamMin=[]  KtParamMax=[]  KbOutMin=[]  KbOutMax=[]  KtOutMin=[]  KtOutMax=[]  IntegratorOutMin=[]  IntegratorOutMax=[]  FilterOutMin=[]  FilterOutMax=[]  SumI1OutMin=[]  SumI1OutMax=[]  SumI2OutMin=[]  SumI2OutMax=[]  SumI3OutMin=[]  SumI3OutMax=[]  SumI4OutMin=[]  SumI4OutMax=[]  SumDOutMin=[]  SumDOutMax=[]  DifferentiatorOutMin=[]  DifferentiatorOutMax=[]  FilterDiffOutCoefMin=[]  FilterDiffOutCoefMax=[]  ReciprocalOutMin=[]  ReciprocalOutMax=[]  SumDenOutMin=[]  SumDenOutMax=[]  SumNumOutMin=[]  SumNumOutMax=[]  DivideOutMin=[]  DivideOutMax=[]  UdiffTsProdOutMin=[]  UdiffTsProdOutMax=[]  NTsProdOutMin=[]  NTsProdOutMax=[]  UintegralTsProdOutMin=[]  UintegralTsProdOutMax=[]  UngainTsProdOutMin=[]  UngainTsProdOutMax=[]  ClampingZeroOutDataTypeStr=Inherit: Inherit via back propagation  ClampingZeroOutMin=[]  ClampingZeroOutMax=[]  FilterDenConstantOutDataTypeStr=Inherit: Inherit via back propagation  FilterDenConstantOutMin=[]  FilterDenConstantOutMax=[]  PCopyOutDataTypeStr=Inherit: Inherit via back propagation  PCopyOutMin=[]  PCopyOutMax=[]  NCopyOutDataTypeStr=Inherit: Inherit via back propagation  NCopyOutMin=[]  NCopyOutMax=[]  IntegratorContinuousStateAttributes=''  IntegratorStateMustResolveToSignalObject=off  IntegratorRTWStateStorageClass=Auto  FilterContinuousStateAttributes=''  FilterStateMustResolveToSignalObject=off  FilterRTWStateStorageClass=Auto  ParallelPVariant=InternalParameters  IdealPVariant=Disabled  IVariant=Disabled  DVariant=InternalParameters  IntegratorVariant=Disabled  SatVariant=Disabled  AWVariant=Disabled  PCopyVariant=Disabled  TRVariant=Disabled  FdbkBlocksVariant=Forward  IdealPFdbkVariant=Disabled  SatFdbkVariant=Disabled  DerivativeFilterVariant=ForwardEulerFilter  NVariant=InternalParameters  NCopyVariant=Disabled  FilterICVariant=InternalICsFilter  IntegratorICVariant=Disabled  ExternalResetVariant=Disabled  TRSumVariant=Passthrough  SumFdbkVariant=Disabled  SumVariant=Sum_PD  TsampFilterVariant=InternalTs  TsampNgainVariant=Passthrough  TsampIntegralVariant=Disabled_SignalSpec  ExternalSaturationOutDataTypeStr=Inherit: Same as second input
  Sum : Sum  Inputs=|+-
  tau_psi : Outport
  wires:
  Sum/1 -> PID Controller/1
  state_estimates/1 -> Bus Selector/1
  Bus Selector/1 -> Sum/2  "<yaw>"
  PID Controller/1 -> tau_psi/1
  Bus Selector1/1 -> Sum/1  "<yaw>"
  heading_sp/1 -> Bus Selector1/1  "heading_sp"

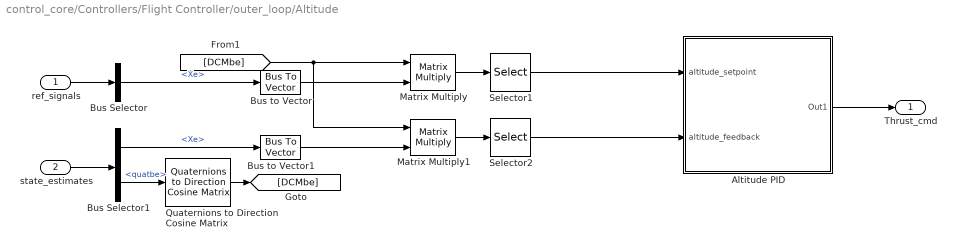
== system control_core/Controllers/Flight Controller/outer_loop/Altitude ==
  ref_signals : Inport  OutDataTypeStr=Bus: reference_signals
  state_estimates : Inport  Port=2  OutDataTypeStr=Bus: state_estimates
  Altitude PID : Subsystem
  Bus Selector : BusSelector  OutputSignals=Xe
  Bus Selector1 : BusSelector  OutputSignals=Xe,quatbe
  Bus to Vector : BusToVector
  Bus to Vector1 : BusToVector
  Matrix Multiply : Product  Multiplication=Matrix(*)
  Matrix Multiply1 : Product  Multiplication=Matrix(*)
  Quaternions to Direction Cosine Matrix : sharedtransform/Quaternions to  Direction Cosine Matrix  aMode=aMode
      settings: LibrarySourceBlock=|
      | aerolibtransform2/Quaternions to
      | Direction Cosine Matrix
  Selector1 : Selector  InputPortWidth=3  IndexOptions=Index vector (dialog)  Indices=[3]  OutputSizes=1
  Selector2 : Selector  InputPortWidth=3  IndexOptions=Index vector (dialog)  Indices=[3]  OutputSizes=1
  Thrust_cmd : Outport
  wires:
  Altitude PID/1(Out1) -> Thrust_cmd/1
  Selector2/1 -> Altitude PID/2(altitude_feedback)
  Selector1/1 -> Altitude PID/1(altitude_setpoint)
  Matrix Multiply/1 -> Selector1/1
  Matrix Multiply1/1 -> Selector2/1
  [DCMbe] -> Matrix Multiply/1, Matrix Multiply1/1
  Bus Selector1/2 -> Quaternions to Direction Cosine Matrix/1  "<quatbe>"
  state_estimates/1 -> Bus Selector1/1
  ref_signals/1 -> Bus Selector/1
  Bus Selector/1 -> Bus to Vector/1  "<Xe>"
  Bus Selector1/1 -> Bus to Vector1/1  "<Xe>"
  Bus to Vector/1 -> Matrix Multiply/2
  Bus to Vector1/1 -> Matrix Multiply1/2
  Quaternions to Direction Cosine Matrix/1 -> [DCMbe]

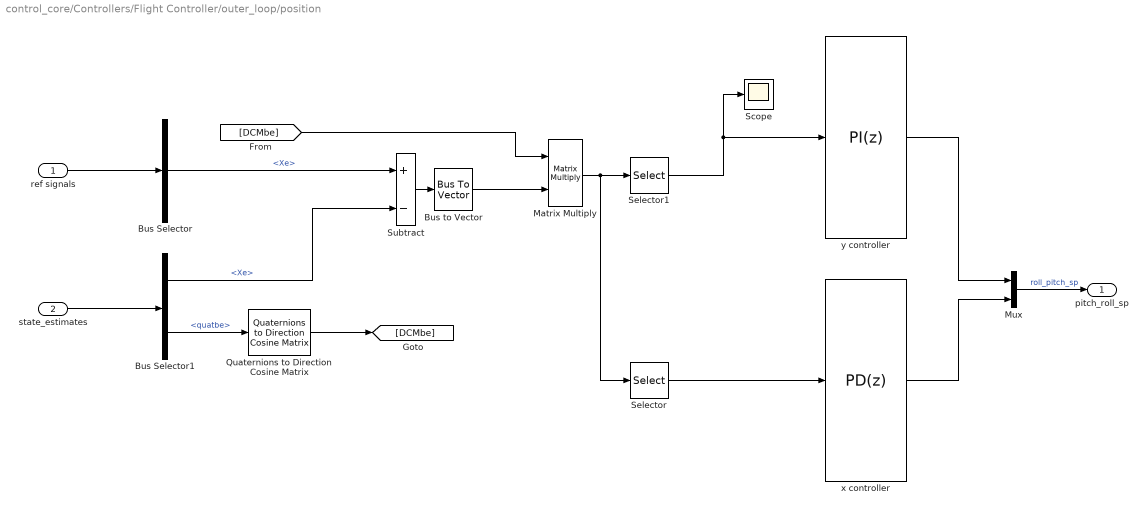
== system control_core/Controllers/Flight Controller/outer_loop/position ==
  ref signals : Inport  OutDataTypeStr=Bus: reference_signals
  state_estimates : Inport  Port=2  OutDataTypeStr=Bus: state_estimates
  Bus Selector : BusSelector  OutputSignals=Xe
  Bus Selector1 : BusSelector  OutputSignals=Xe,quatbe
  Bus to Vector : BusToVector
  Matrix Multiply : Product  Multiplication=Matrix(*)
  Mux : Mux  Inputs=2
  Quaternions to Direction Cosine Matrix : sharedtransform/Quaternions to  Direction Cosine Matrix  aMode=aMode
      settings: LibrarySourceBlock=|
      | aerolibtransform2/Quaternions to
      | Direction Cosine Matrix
  Scope : Scope
  Selector : Selector  InputPortWidth=3  IndexOptions=Index vector (dialog)  Indices=[1]  OutputSizes=1
  Selector1 : Selector  InputPortWidth=3  IndexOptions=Index vector (dialog)  Indices=[2]  OutputSizes=1
  Subtract : Sum  Inputs=+-
  x controller : slpidlib/PID Controller  Controller=PD  Form=Parallel  TimeDomain=Discrete-time  UseExternalTs=off  SampleTime=-1  IntegratorMethod=Forward Euler  FilterMethod=Forward Euler  ControllerParametersSource=internal  P=-0.0205622316535753  I=.000001  UseKiTs=off  D=0  N=100  UseFilter=on  TunerSelectOption=Transfer Function Based (PID Tuner App)  InitialConditionSource=internal  InitialConditionForIntegrator=0  InitialConditionForFilter=0  DifferentiatorICPrevScaledInput=0  ExternalReset=none  TrackingMode=off  Kt=1  LimitOutput=off  SatLimitsSource=internal  UpperSaturationLimit=inf  LowerSaturationLimit=-inf  LinearizeAsGain=on  AntiWindupMode=clamping  Kb=1  LimitIntegrator=off  UpperIntegratorSaturationLimit=inf  LowerIntegratorSaturationLimit=-inf  POutMin=[]  POutMax=[]  IOutMin=[]  IOutMax=[]  DOutMin=[]  DOutMax=[]  NOutMin=[]  NOutMax=[]  SumOutMin=[]  SumOutMax=[]  SaturationOutMin=[]  SaturationOutMax=[]  PParamMin=[]  PParamMax=[]  IParamMin=[]  IParamMax=[]  DParamMin=[]  DParamMax=[]  NParamMin=[]  NParamMax=[]  KbParamMin=[]  KbParamMax=[]  KtParamMin=[]  KtParamMax=[]  KbOutMin=[]  KbOutMax=[]  KtOutMin=[]  KtOutMax=[]  IntegratorOutMin=[]  IntegratorOutMax=[]  FilterOutMin=[]  FilterOutMax=[]  SumI1OutMin=[]  SumI1OutMax=[]  SumI2OutMin=[]  SumI2OutMax=[]  SumI3OutMin=[]  SumI3OutMax=[]  SumI4OutMin=[]  SumI4OutMax=[]  SumDOutMin=[]  SumDOutMax=[]  DifferentiatorOutMin=[]  DifferentiatorOutMax=[]  FilterDiffOutCoefMin=[]  FilterDiffOutCoefMax=[]  ReciprocalOutMin=[]  ReciprocalOutMax=[]  SumDenOutMin=[]  SumDenOutMax=[]  SumNumOutMin=[]  SumNumOutMax=[]  DivideOutMin=[]  DivideOutMax=[]  UdiffTsProdOutMin=[]  UdiffTsProdOutMax=[]  NTsProdOutMin=[]  NTsProdOutMax=[]  UintegralTsProdOutMin=[]  UintegralTsProdOutMax=[]  UngainTsProdOutMin=[]  UngainTsProdOutMax=[]  ClampingZeroOutDataTypeStr=Inherit: Inherit via back propagation  ClampingZeroOutMin=[]  ClampingZeroOutMax=[]  FilterDenConstantOutDataTypeStr=Inherit: Inherit via back propagation  FilterDenConstantOutMin=[]  FilterDenConstantOutMax=[]  PCopyOutDataTypeStr=Inherit: Inherit via back propagation  PCopyOutMin=[]  PCopyOutMax=[]  NCopyOutDataTypeStr=Inherit: Inherit via back propagation  NCopyOutMin=[]  NCopyOutMax=[]  IntegratorContinuousStateAttributes=''  IntegratorStateMustResolveToSignalObject=off  IntegratorRTWStateStorageClass=Auto  FilterContinuousStateAttributes=''  FilterStateMustResolveToSignalObject=off  FilterRTWStateStorageClass=Auto  ParallelPVariant=InternalParameters  IdealPVariant=Disabled  IVariant=Disabled  DVariant=InternalParameters  IntegratorVariant=Disabled  SatVariant=Disabled  AWVariant=Disabled  PCopyVariant=Disabled  TRVariant=Disabled  FdbkBlocksVariant=Forward  IdealPFdbkVariant=Disabled  SatFdbkVariant=Disabled  DerivativeFilterVariant=ForwardEulerFilter  NVariant=InternalParameters  NCopyVariant=Disabled  FilterICVariant=InternalICsFilter  IntegratorICVariant=Disabled  ExternalResetVariant=Disabled  TRSumVariant=Passthrough  SumFdbkVariant=Disabled  SumVariant=Sum_PD  TsampFilterVariant=InternalTs  TsampNgainVariant=Passthrough  TsampIntegralVariant=Disabled_SignalSpec  ExternalSaturationOutDataTypeStr=Inherit: Same as second input
  y controller : slpidlib/PID Controller  Controller=PI  Form=Parallel  TimeDomain=Discrete-time  UseExternalTs=off  SampleTime=-1  IntegratorMethod=Forward Euler  FilterMethod=Forward Euler  ControllerParametersSource=internal  P=0.0214287173644059  I=8.55230649524744e-05  UseKiTs=off  D=0  N=100  UseFilter=on  TunerSelectOption=Transfer Function Based (PID Tuner App)  InitialConditionSource=internal  InitialConditionForIntegrator=0  InitialConditionForFilter=0  DifferentiatorICPrevScaledInput=0  ExternalReset=none  TrackingMode=off  Kt=1  LimitOutput=off  SatLimitsSource=internal  UpperSaturationLimit=inf  LowerSaturationLimit=-inf  LinearizeAsGain=on  AntiWindupMode=clamping  Kb=1  LimitIntegrator=off  UpperIntegratorSaturationLimit=inf  LowerIntegratorSaturationLimit=-inf  POutMin=[]  POutMax=[]  IOutMin=[]  IOutMax=[]  DOutMin=[]  DOutMax=[]  NOutMin=[]  NOutMax=[]  SumOutMin=[]  SumOutMax=[]  SaturationOutMin=[]  SaturationOutMax=[]  PParamMin=[]  PParamMax=[]  IParamMin=[]  IParamMax=[]  DParamMin=[]  DParamMax=[]  NParamMin=[]  NParamMax=[]  KbParamMin=[]  KbParamMax=[]  KtParamMin=[]  KtParamMax=[]  KbOutMin=[]  KbOutMax=[]  KtOutMin=[]  KtOutMax=[]  IntegratorOutMin=[]  IntegratorOutMax=[]  FilterOutMin=[]  FilterOutMax=[]  SumI1OutMin=[]  SumI1OutMax=[]  SumI2OutMin=[]  SumI2OutMax=[]  SumI3OutMin=[]  SumI3OutMax=[]  SumI4OutMin=[]  SumI4OutMax=[]  SumDOutMin=[]  SumDOutMax=[]  DifferentiatorOutMin=[]  DifferentiatorOutMax=[]  FilterDiffOutCoefMin=[]  FilterDiffOutCoefMax=[]  ReciprocalOutMin=[]  ReciprocalOutMax=[]  SumDenOutMin=[]  SumDenOutMax=[]  SumNumOutMin=[]  SumNumOutMax=[]  DivideOutMin=[]  DivideOutMax=[]  UdiffTsProdOutMin=[]  UdiffTsProdOutMax=[]  NTsProdOutMin=[]  NTsProdOutMax=[]  UintegralTsProdOutMin=[]  UintegralTsProdOutMax=[]  UngainTsProdOutMin=[]  UngainTsProdOutMax=[]  ClampingZeroOutDataTypeStr=Inherit: Inherit via back propagation  ClampingZeroOutMin=[]  ClampingZeroOutMax=[]  FilterDenConstantOutDataTypeStr=Inherit: Inherit via back propagation  FilterDenConstantOutMin=[]  FilterDenConstantOutMax=[]  PCopyOutDataTypeStr=Inherit: Inherit via back propagation  PCopyOutMin=[]  PCopyOutMax=[]  NCopyOutDataTypeStr=Inherit: Inherit via back propagation  NCopyOutMin=[]  NCopyOutMax=[]  IntegratorContinuousStateAttributes=''  IntegratorStateMustResolveToSignalObject=off  IntegratorRTWStateStorageClass=Auto  FilterContinuousStateAttributes=''  FilterStateMustResolveToSignalObject=off  FilterRTWStateStorageClass=Auto  ParallelPVariant=InternalParameters  IdealPVariant=Disabled  IVariant=InternalParameters  DVariant=Disabled  IntegratorVariant=Discrete  SatVariant=Disabled  AWVariant=Passthrough  PCopyVariant=Disabled  TRVariant=Disabled  FdbkBlocksVariant=Forward  IdealPFdbkVariant=Disabled  SatFdbkVariant=Disabled  DerivativeFilterVariant=Disabled  NVariant=Disabled  NCopyVariant=Disabled_SignalSpec  FilterICVariant=Disabled  IntegratorICVariant=InternalICs  ExternalResetVariant=Disabled  TRSumVariant=Passthrough  SumFdbkVariant=Disabled  SumVariant=Sum_PI  TsampFilterVariant=InternalTs  TsampNgainVariant=Passthrough  TsampIntegralVariant=Passthrough  ExternalSaturationOutDataTypeStr=Inherit: Same as second input
  pitch_roll_sp : Outport
  wires:
  y controller/1 -> Mux/1
  x controller/1 -> Mux/2
  Mux/1 -> pitch_roll_sp/1  "roll_pitch_sp"
  Selector1/1 -> Scope/1, y controller/1
  Selector/1 -> x controller/1
  Matrix Multiply/1 -> Selector/1, Selector1/1
  Bus Selector1/2 -> Quaternions to Direction Cosine Matrix/1  "<quatbe>"
  [DCMbe] -> Matrix Multiply/1
  Bus Selector1/1 -> Subtract/2  "<Xe>"
  Bus Selector/1 -> Subtract/1  "<Xe>"
  state_estimates/1 -> Bus Selector1/1
  ref signals/1 -> Bus Selector/1
  Subtract/1 -> Bus to Vector/1
  Bus to Vector/1 -> Matrix Multiply/2
  Quaternions to Direction Cosine Matrix/1 -> [DCMbe]

== system control_core/visualization/simulink_3D/Simulink 3D/Axes to VR Axes ==
  Xe : Inport
  Constant : Constant  Value=50
  Constant1 : Constant  Value=.0460
  Constant2 : Constant  Value=95
  Demux : Demux  Outputs=3
      settings: DisplayOption=none
  Mux : Mux  Inputs=3
  Sum : Sum  Inputs=|++
  Sum1 : Sum  Inputs=|++
  Sum2 : Sum  Inputs=|++
  rad-->deg1 : Gain  Gain=-1  SaturateOnIntegerOverflow=on  OutDataTypeStr=Inherit: Same as input  ParamDataTypeStr=Inherit: Same as input
  Xe VR : Outport  VectorParamsAs1DForOutWhenUnconnected=off
  wires:
  Xe/1 -> Demux/1
  Demux/3 -> rad-->deg1/1
  Mux/1 -> Xe VR/1
  Demux/1 -> Sum/1
  Demux/2 -> Sum1/1
  rad-->deg1/1 -> Sum2/1
  Constant/1 -> Sum/2
  Sum/1 -> Mux/1
  Constant2/1 -> Sum1/2
  Constant1/1 -> Sum2/2
  Sum1/1 -> Mux/3
  Sum2/1 -> Mux/2

== system control_core/visualization/simulink_3D/Simulink 3D/Axes to VR Axes Camera Chase ==
  Xe : Inport
  Demux : Demux  Outputs=3
      settings: DisplayOption=none
  Mux : Mux  Inputs=3
  rad-->deg1 : Gain  Gain=-1  SaturateOnIntegerOverflow=on  OutDataTypeStr=Inherit: Same as input  ParamDataTypeStr=Inherit: Same as input
  Xe VR : Outport  VectorParamsAs1DForOutWhenUnconnected=off
  wires:
  Xe/1 -> Demux/1
  Demux/1 -> Mux/1
  Demux/3 -> rad-->deg1/1
  Mux/1 -> Xe VR/1
  rad-->deg1/1 -> Mux/2
  Demux/2 -> Mux/3

== system control_core/visualization/simulink_3D/Simulink 3D/Axes to VR Axes Camera Iso ==
  Xe : Inport
  Demux : Demux  Outputs=3
      settings: DisplayOption=none
  Mux : Mux  Inputs=3
  rad-->deg1 : Gain  Gain=-1  SaturateOnIntegerOverflow=on  OutDataTypeStr=Inherit: Same as input  ParamDataTypeStr=Inherit: Same as input
  Xe VR : Outport  VectorParamsAs1DForOutWhenUnconnected=off
  wires:
  Demux/2 -> Mux/3
  rad-->deg1/1 -> Mux/2
  Mux/1 -> Xe VR/1
  Demux/3 -> rad-->deg1/1
  Demux/1 -> Mux/1
  Xe/1 -> Demux/1

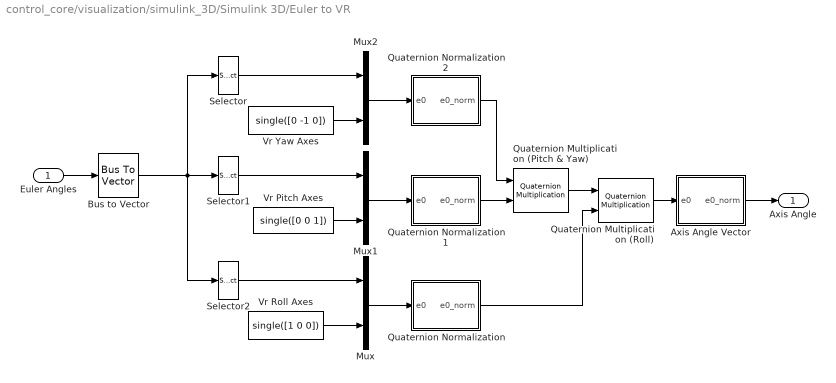
== system control_core/visualization/simulink_3D/Simulink 3D/Euler to VR ==
  Euler Angles : Inport
  Axis Angle Vector : Subsystem
  Bus to Vector : BusToVector
  Mux : Mux  Inputs=2
  Mux1 : Mux  Inputs=2
  Mux2 : Mux  Inputs=2
  Quaternion Multiplication (Pitch & Yaw) : aerolibutil/Quaternion Multiplication
  Quaternion Multiplication (Roll) : aerolibutil/Quaternion Multiplication
  Quaternion Normalization : Subsystem
  Quaternion Normalization1 : Subsystem
  Quaternion Normalization2 : Subsystem
  Selector : Selector  InputPortWidth=3  IndexOptions=Index vector (dialog)  Indices=[3]  OutputSizes=1
  Selector1 : Selector  InputPortWidth=3  IndexOptions=Index vector (dialog)  Indices=[2]  OutputSizes=1
  Selector2 : Selector  InputPortWidth=3  IndexOptions=Index vector (dialog)  Indices=[1]  OutputSizes=1
  Vr Pitch Axes : Constant  Value=single([0 0 1])
  Vr Roll Axes : Constant  Value=single([1 0 0])
  Vr Yaw Axes : Constant  Value=single([0 -1 0])
  Axis Angle : Outport  VectorParamsAs1DForOutWhenUnconnected=off
  wires:
  Quaternion Multiplication (Roll)/1 -> Axis Angle Vector/1(e0)
  Axis Angle Vector/1(e0_norm) -> Axis Angle/1
  Quaternion Normalization/1(e0_norm) -> Quaternion Multiplication (Roll)/2
  Quaternion Normalization2/1(e0_norm) -> Quaternion Multiplication (Pitch & Yaw)/1
  Quaternion Normalization1/1(e0_norm) -> Quaternion Multiplication (Pitch & Yaw)/2
  Mux2/1 -> Quaternion Normalization2/1(e0)
  Mux1/1 -> Quaternion Normalization1/1(e0)
  Mux/1 -> Quaternion Normalization/1(e0)
  Selector/1 -> Mux2/1
  Vr Yaw Axes/1 -> Mux2/2
  Selector1/1 -> Mux1/1
  Vr Pitch Axes/1 -> Mux1/2
  Selector2/1 -> Mux/1
  Vr Roll Axes/1 -> Mux/2
  Euler Angles/1 -> Bus to Vector/1
  Quaternion Multiplication (Pitch & Yaw)/1 -> Quaternion Multiplication (Roll)/1
  Bus to Vector/1 -> Selector2/1, Selector1/1, Selector/1

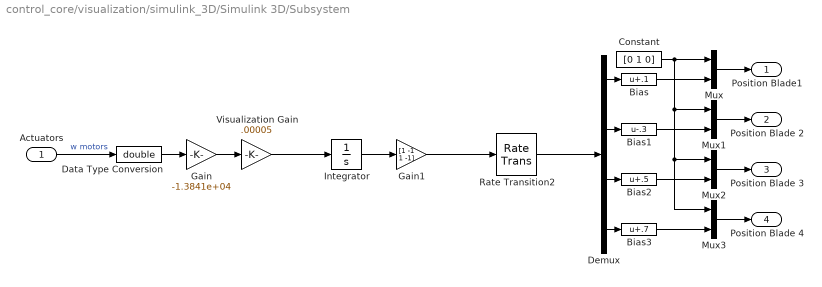
== system control_core/visualization/simulink_3D/Simulink 3D/Subsystem ==
  Actuators : Inport
  Bias : Bias  Bias=.1  SaturateOnIntegerOverflow=off
  Bias1 : Bias  Bias=-.3  SaturateOnIntegerOverflow=off
  Bias2 : Bias  Bias=.5  SaturateOnIntegerOverflow=off
  Bias3 : Bias  Bias=.7  SaturateOnIntegerOverflow=off
  Constant : Constant  Value=[0 1 0]
  Data Type Conversion : DataTypeConversion  OutDataTypeStr=double  SaturateOnIntegerOverflow=off  RndMeth=Floor
  Demux : Demux
  Gain : Gain  Gain=-1.3841e+04
  Gain1 : Gain  Gain=[1 -1 1 -1]
  Integrator : Integrator  InitialCondition="[.1  .2 -.3 -.4]"  WrapState=on  WrappedStateUpperValue=2*pi  WrappedStateLowerValue=-2*pi
  Mux{,1..3} (4 alike) : Mux  Inputs=2
  Rate Transition2 : RateTransition
  Visualization Gain : Gain  Gain=.00005
  Position Blade1 : Outport  VectorParamsAs1DForOutWhenUnconnected=off
  Position Blade 2 : Outport  Port=2  VectorParamsAs1DForOutWhenUnconnected=off
  Position Blade 3 : Outport  Port=3  VectorParamsAs1DForOutWhenUnconnected=off
  Position Blade 4 : Outport  Port=4  VectorParamsAs1DForOutWhenUnconnected=off
  wires:
  Bias3/1 -> Mux3/2
  Mux3/1 -> Position Blade 4/1
  Bias1/1 -> Mux1/2
  Bias2/1 -> Mux2/2
  Demux/2 -> Bias1/1
  Visualization Gain/1 -> Integrator/1
  Constant/1 -> Mux3/1, Mux2/1, Mux1/1, Mux/1
  Mux1/1 -> Position Blade 2/1
  Mux2/1 -> Position Blade 3/1
  Data Type Conversion/1 -> Gain/1
  Mux/1 -> Position Blade1/1
  Gain/1 -> Visualization Gain/1
  Demux/3 -> Bias2/1
  Bias/1 -> Mux/2
  Actuators/1 -> Data Type Conversion/1  "w motors"
  Demux/4 -> Bias3/1
  Rate Transition2/1 -> Demux/1
  Demux/1 -> Bias/1
  Integrator/1 -> Gain1/1
  Gain1/1 -> Rate Transition2/1

== system control_core/Controllers/Flight Controller/outer_loop/Altitude/Altitude PID ==
  altitude_setpoint : Inport
  altitude_feedback : Inport  Port=2
  Constant : Constant  Value=-g*mass
  PID Controller : slpidlib/PID Controller  Controller=PD  Form=Parallel  TimeDomain=Discrete-time  UseExternalTs=off  SampleTime=-1  IntegratorMethod=Forward Euler  FilterMethod=Forward Euler  ControllerParametersSource=internal  P=0.391711979722748  I=0  UseKiTs=off  D=0.101719151159153  N=0.643160901514191  UseFilter=on  TunerSelectOption=Transfer Function Based (PID Tuner App)  InitialConditionSource=internal  InitialConditionForIntegrator=0  InitialConditionForFilter=0  DifferentiatorICPrevScaledInput=0  ExternalReset=none  TrackingMode=off  Kt=1  LimitOutput=off  SatLimitsSource=internal  UpperSaturationLimit=inf  LowerSaturationLimit=-inf  LinearizeAsGain=on  AntiWindupMode=clamping  Kb=1  LimitIntegrator=off  UpperIntegratorSaturationLimit=inf  LowerIntegratorSaturationLimit=-inf  POutMin=[]  POutMax=[]  IOutMin=[]  IOutMax=[]  DOutMin=[]  DOutMax=[]  NOutMin=[]  NOutMax=[]  SumOutMin=[]  SumOutMax=[]  SaturationOutMin=[]  SaturationOutMax=[]  PParamMin=[]  PParamMax=[]  IParamMin=[]  IParamMax=[]  DParamMin=[]  DParamMax=[]  NParamMin=[]  NParamMax=[]  KbParamMin=[]  KbParamMax=[]  KtParamMin=[]  KtParamMax=[]  KbOutMin=[]  KbOutMax=[]  KtOutMin=[]  KtOutMax=[]  IntegratorOutMin=[]  IntegratorOutMax=[]  FilterOutMin=[]  FilterOutMax=[]  SumI1OutMin=[]  SumI1OutMax=[]  SumI2OutMin=[]  SumI2OutMax=[]  SumI3OutMin=[]  SumI3OutMax=[]  SumI4OutMin=[]  SumI4OutMax=[]  SumDOutMin=[]  SumDOutMax=[]  DifferentiatorOutMin=[]  DifferentiatorOutMax=[]  FilterDiffOutCoefMin=[]  FilterDiffOutCoefMax=[]  ReciprocalOutMin=[]  ReciprocalOutMax=[]  SumDenOutMin=[]  SumDenOutMax=[]  SumNumOutMin=[]  SumNumOutMax=[]  DivideOutMin=[]  DivideOutMax=[]  UdiffTsProdOutMin=[]  UdiffTsProdOutMax=[]  NTsProdOutMin=[]  NTsProdOutMax=[]  UintegralTsProdOutMin=[]  UintegralTsProdOutMax=[]  UngainTsProdOutMin=[]  UngainTsProdOutMax=[]  ClampingZeroOutDataTypeStr=Inherit: Inherit via back propagation  ClampingZeroOutMin=[]  ClampingZeroOutMax=[]  FilterDenConstantOutDataTypeStr=Inherit: Inherit via back propagation  FilterDenConstantOutMin=[]  FilterDenConstantOutMax=[]  PCopyOutDataTypeStr=Inherit: Inherit via back propagation  PCopyOutMin=[]  PCopyOutMax=[]  NCopyOutDataTypeStr=Inherit: Inherit via back propagation  NCopyOutMin=[]  NCopyOutMax=[]  IntegratorContinuousStateAttributes=''  IntegratorStateMustResolveToSignalObject=off  IntegratorRTWStateStorageClass=Auto  FilterContinuousStateAttributes=''  FilterStateMustResolveToSignalObject=off  FilterRTWStateStorageClass=Auto  ParallelPVariant=InternalParameters  IdealPVariant=Disabled  IVariant=Disabled  DVariant=InternalParameters  IntegratorVariant=Disabled  SatVariant=Disabled  AWVariant=Disabled  PCopyVariant=Disabled  TRVariant=Disabled  FdbkBlocksVariant=Forward  IdealPFdbkVariant=Disabled  SatFdbkVariant=Disabled  DerivativeFilterVariant=ForwardEulerFilter  NVariant=InternalParameters  NCopyVariant=Disabled  FilterICVariant=InternalICsFilter  IntegratorICVariant=Disabled  ExternalResetVariant=Disabled  TRSumVariant=Passthrough  SumFdbkVariant=Disabled  SumVariant=Sum_PD  TsampFilterVariant=InternalTs  TsampNgainVariant=Passthrough  TsampIntegralVariant=Disabled_SignalSpec  ExternalSaturationOutDataTypeStr=Inherit: Same as second input
  Sum : Sum  Inputs=|+-
  Sum1 : Sum  Inputs=|++
  Out1 : Outport
  wires:
  altitude_setpoint/1 -> Sum/1
  Sum1/1 -> Out1/1
  altitude_feedback/1 -> Sum/2
  Constant/1 -> Sum1/2
  PID Controller/1 -> Sum1/1
  Sum/1 -> PID Controller/1
